simulink model "L68"  (Simulink 8.0)
settings: Solver=ode45  StartTime=0.0  StopTime=30.0  RelTol=1e-3
values from neighbouring files (symbols this model uses):
  A = [0 1 0; 0 0 1; -22 -27 -33]    [t6.m]
  B = [0;0;14]    [t6.m]
  C = [1 0 0]    [t6.m]
settings Model: Creator=12105774  LastModifiedBy=mebuffet
settings DebuggingCC: FrameProcessingCompatibilityMsg=error
settings CodeAppCC: CustomSymbolStrType=$N$R$M_T
settings GRTTargetCC: CodeReplacementLibrary=C89/C90 (ANSI)

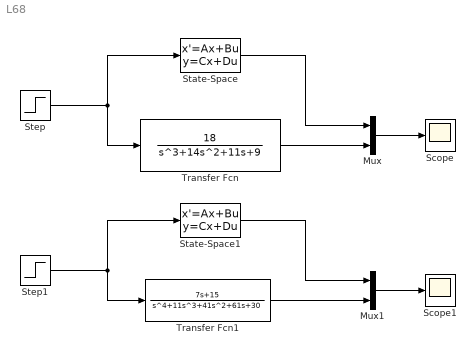
== system L68 ==
  Mux : Mux  Inputs=2
  Mux1 : Mux  Inputs=2
  Scope : Scope
      settings: TimeRange=auto  ShowLegends=on  MaxDataPoints=5000  SaveToWorkspace=off  SaveName=ScopeData  YMin=-10  YMax=10  SampleTime=-1
  Scope1 : Scope
      settings: TimeRange=auto  ShowLegends=on  MaxDataPoints=5000  SaveToWorkspace=off  YMin=-10  YMax=10  SampleTime=-1
  State-Space : StateSpace  A=A  B=B  C=C  D=0  X0=0
  State-Space1 : StateSpace  A=[0 1 0 0; 0 0 1 0; 0 0 0 1; -30 -61 -41 -11]  B=[0; 0; 0; 1]  C=[15 7 0 0]  D=0  X0=0
  Step : Step  SampleTime=0
  Step1 : Step  SampleTime=0
  Transfer Fcn : TransferFcn  Numerator=[18]  Denominator=[1 14 11 9]
  Transfer Fcn1 : TransferFcn  Numerator=[7 15]  Denominator=[1 11 41 61 30]
  wires:
  Transfer Fcn/1 -> Mux/2
  State-Space/1 -> Mux/1
  Step/1 -> Transfer Fcn/1, State-Space/1
  Mux/1 -> Scope/1
  Transfer Fcn1/1 -> Mux1/2
  State-Space1/1 -> Mux1/1
  Step1/1 -> Transfer Fcn1/1, State-Space1/1
  Mux1/1 -> Scope1/1
